simulink model "doc_carrier"  (Simulink 6.0)
settings: Solver=ode45  StartTime=0.0  StopTime=inf  RelTol=1e-3
undefined symbols (not defined in the file): slcm
libraries: commsink2 x2, commdigbbndpm2 x2, commfilt2 x2, commchan2 x1, commphrec2 x1, commrflib2 x1, commrandsrc2 x1, commtimrec2 x1, dspsigops x1
settings Model: Creator=arodrigu  LastModifiedBy=agaltman  ProdHWDeviceType=Specified  UpdateModelReferenceTargets=IfOutOfDate
settings DataIOCC: SaveOutput=off  SaveTime=off  SignalLoggingName=logsOut
settings DebuggingCC: CheckExecutionContextPreStartOutputMsg=on  CheckExecutionContextRuntimeOutputMsg=on  SolverPrmCheckMsg=none  InheritedTsInSrcMsg=none
settings HardwareCC: ProdHWDeviceType=Specified
settings ModelReferenceCC: UpdateModelReferenceTargets=IfOutOfDate
settings CodeAppCC: MangleLength=5
settings GRTTargetCC: UtilityFuncGeneration=Automatic  LifeSpan=inf
settings SFSimCC: SFSimApplyToAllLibs=on  SFSimBuildMode=Incremental

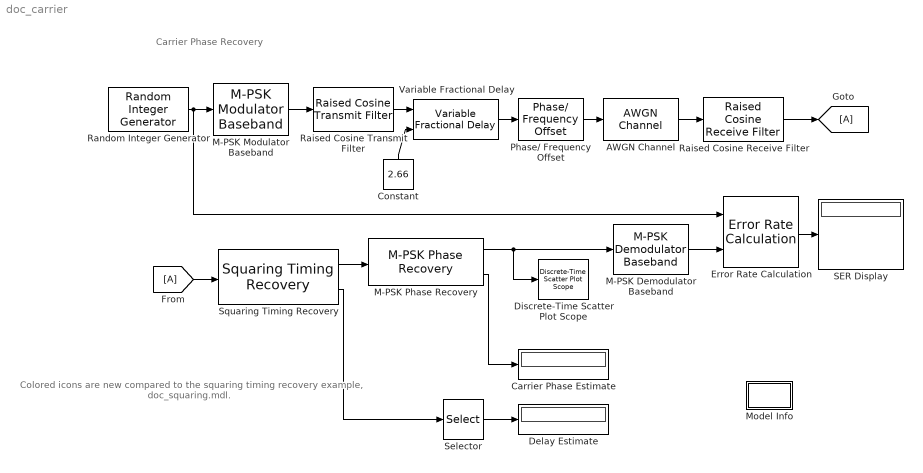
== system doc_carrier ==
  note: Carrier Phase Recovery
  note: Colored icons are new compared
      | to the squaring timing recovery
      | example, doc_squaring.mdl.
  AWGN Channel : commchan2/AWGN Channel  seed=67  noiseMode="Signal to noise ratio  (SNR)"  EbNodB=10  EsNodB=10  SNRdB=40  bitsPerSym=1  Ps=1  Tsym=1  variance=1
  Carrier Phase Estimate : Display
  Constant : Constant  Orientation=up  Value=2.66
  Delay Estimate : Display
  Discrete-Time Scatter Plot Scope : commsink2/Discrete-Time Scatter Plot Scope  Tag=ScatterPlot  sampPerSymb=1  offsetEye=0  numTraces=400  numNewFrames=10  LineMarkers=.  LineColors=b  fading=on  render=on  AxisGrid=on  xMin=-1.5  xMax=1.5  yMin=-1.5  yMax=1.5  inphaseLabel=In-phase Amplitude  quadratureLabel=Quadrature Amplitude  openScopeAtSimStart=on  FrameNumber=off  FigPos=[60 447 400 400]  figTitle=Scatter Plot  numLinesMax=8  block_type_=scatter
  Error Rate Calculation : commsink2/Error Rate Calculation  N=2*4  st_delay=500  cp_mode=Entire frame  subframe=[]  PMode=Port  WsName=ErrorVec  RsMode2=off  stop=off  numErr=100  maxBits=1e6
  M-PSK Demodulator Baseband : commdigbbndpm2/M-PSK Demodulator Baseband  M=16  OutType=Integer  Dec=Binary  Ph=0  numSamp=1
  M-PSK Modulator Baseband : commdigbbndpm2/M-PSK Modulator Baseband  M=16  InType=Integer  Enc=Binary  Ph=0  numSamp=1
  M-PSK Phase Recovery : commphrec2/M-PSK Phase Recovery  M=16  intPeriod=500
  Model Info : Subsystem  LoadFcn=slcm LoadBlock;  InitFcn=slcm('UpdateAllCMBlocksInThisModelInit')  EnableExecutionContextPropagation=on  mask(CMBlock){InitialSaveTempField=, InitialBlockCM=None, BlockCM=None, Frame=on, SaveTempField=, DisplayStringWithTags=Info, MaskDisplayString=Info, HorizontalTextAlignment=Center, LeftAlignmentValue=0.5, SourceBlockDiagram=doc_carrier, TagMaxNumber=20, CMTag1=, CMTag2=, CMTag3=, CMTag4=, CMTag5=, CMTag6=, CMTag7=, CMTag8=, CMTag9=, CMTag10=, CMTag11=, CMTag12=, CMTag13=, CMTag14=, CMTag15=, CMTag16=, CMTag17=, CMTag18=, CMTag19=, CMTag20=}
      mask help: This block allows revision control information to be displayed within the model.
      settings: CopyFcn=slcm CopyBlock;  DeleteFcn=slcm Cancel;  PostSaveFcn=slcm('UpdateAllCMBlocksInThisModel')  NameChangeFcn=slcm Rename;  OpenFcn=commdemohelp;
      mask Display: text(str2num(LeftAlignmentValue), 0.5, MaskDisplayString, 'HorizontalAlignment', HorizontalTextAlignment)
  Phase/ Frequency Offset : commrflib2/Phase// Frequency Offset  freqOffset=0  phaseOffset=10
  Raised Cosine Receive Filter : commfilt2/Raised Cosine Receive Filter  filtType=Square root  N=8  D=4  R=0.2  sampMode=Frame-based  rateMode=None  downFactor=8  downOffset=0  checkGain=Normalized  filterGain=1  checkCoeff=off  variableName=rcRxFilt  launchFVT=off
  Raised Cosine Transmit Filter : commfilt2/Raised Cosine Transmit Filter  filtType=Square root  D=4  R=0.2  sampMode=Frame-based  N=8  checkGain=Normalized  filterGain=1  checkCoeff=off  variableName=rcTxFilt  launchFVT=off
  Random Integer Generator : commrandsrc2/Random Integer Generator  mul=16  seed=37  Ts=1/100  frameBased=on  sampPerFrame=100  orient=off
  SER Display : Display
  Selector : Selector  InputPortWidth=100
  Squaring Timing Recovery : commtimrec2/Squaring Timing Recovery  numSymb=100  sampPerSymb=8
  Variable Fractional Delay : dspsigops/Variable Fractional Delay  mode=Linear Interpolation  dmax=100  L=4  R=10  alpha=1  ic=0
  wires:
  Random Integer Generator/1 -> Error Rate Calculation/1, M-PSK Modulator Baseband/1
  M-PSK Modulator Baseband/1 -> Raised Cosine Transmit Filter/1
  Raised Cosine Receive Filter/1 -> [A]
  AWGN Channel/1 -> Raised Cosine Receive Filter/1
  Constant/1 -> Variable Fractional Delay/2
  Raised Cosine Transmit Filter/1 -> Variable Fractional Delay/1
  Variable Fractional Delay/1 -> Phase/ Frequency Offset/1
  Squaring Timing Recovery/2 -> Selector/1
  Selector/1 -> Delay Estimate/1
  M-PSK Demodulator Baseband/1 -> Error Rate Calculation/2
  Error Rate Calculation/1 -> SER Display/1
  [A] -> Squaring Timing Recovery/1
  Phase/ Frequency Offset/1 -> AWGN Channel/1
  Squaring Timing Recovery/1 -> M-PSK Phase Recovery/1
  M-PSK Phase Recovery/1 -> M-PSK Demodulator Baseband/1, Discrete-Time Scatter Plot Scope/1
  M-PSK Phase Recovery/2 -> Carrier Phase Estimate/1

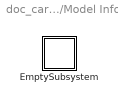
== system doc_carrier/Model Info ==
  EmptySubsystem : Subsystem  EnableExecutionContextPropagation=on

== system doc_carrier/Model Info/EmptySubsystem ==
